simulink model "Torque_Control"  (R2022a)
settings: Solver=FixedStepAuto  StartTime=0.0  StopTime=10.0  RelTol=1e-3
libraries: simulink x9, eeGeneralControl x3
(part 4 of 6)

== system Torque_Control/VDC/Vehicle Dynamics Control Modes/VDC Complete/Optimization SKF & CKF/Subsystem /SKF ==
  Derivative : Inport
  "SKF_Initial " : Inport  Port=2
  SKF_prev : Inport  Port=3
  Cte_SKF : Inport  Port=4
  Action Port : ActionPort  ActionPortLabel=if { }
  Display : Display
  If : If  IfExpression=u1 >=900  ElseIfExpressions=u1 < 900  ShowElse=off
  Merge : Merge
  No spin : Subsystem  TreatAsAtomicUnit=on
  Saturation : Saturate  UpperLimit=1  LowerLimit=0.3
  Spin : Subsystem  TreatAsAtomicUnit=on
  SKF_act : Outport  VectorParamsAs1DForOutWhenUnconnected=off
  wires:
  Merge/1 -> Saturation/1
  Derivative/1 -> If/1, Display/1
  Spin/1(SKF_act1) -> Merge/2
  "SKF_Initial "/1 -> No spin/1(SKF_Initial), Spin/1(SKF_Initial)
  No spin/1(SKF_act0) -> Merge/1
  If/2 -> No spin/Action
  SKF_prev/1 -> No spin/2(SKF_prev), Spin/2(SKF_prev)
  Cte_SKF/1 -> No spin/3(Cte_SKF), Spin/3(Cte_SKF)
  Saturation/1 -> SKF_act/1
  If/1 -> Spin/Action

== system Torque_Control/VDC/Vehicle Dynamics Control Modes/VDC without Longitudinal/Constraints/Acelerating and braking without Regenerative/If Action 1 ==
  Trans_max_dynamic : Inport
  Action Port : ActionPort  ActionPortLabel=if { }
  Trans_limit : Outport  VectorParamsAs1DForOutWhenUnconnected=off
  wires:
  Trans_max_dynamic/1 -> Trans_limit/1

== system Torque_Control/VDC/Vehicle Dynamics Control Modes/VDC without Longitudinal/Constraints/Acelerating and braking without Regenerative/If Action 2 ==
  "Trans_max_static " : Inport
  Action Port : ActionPort  ActionPortLabel=else { }
  Trans_limit : Outport  VectorParamsAs1DForOutWhenUnconnected=off
  wires:
  "Trans_max_static "/1 -> Trans_limit/1

== system Torque_Control/VDC/Vehicle Dynamics Control Modes/VDC without Longitudinal/Constraints/Acelerating and braking without Regenerative/Momentum Z scaled ==
  Tq_RR_Lim : Inport
  Tq_RL_Lim : Inport  Port=2
  Tq_RR_wc : Inport  Port=3
  Tq_RL_wc : Inport  Port=4
  MATLAB Function : MATLAB Function  TreatAsAtomicUnit=on
  TQ_RR : Outport  VectorParamsAs1DForOutWhenUnconnected=off
  TQ_RL : Outport  Port=2  VectorParamsAs1DForOutWhenUnconnected=off
  wires:
  Tq_RL_Lim/1 -> MATLAB Function/2(tq_RL_lim)
  Tq_RR_Lim/1 -> MATLAB Function/1(tq_RR_lim)
  Tq_RR_wc/1 -> MATLAB Function/3(tq_RR_wc)
  Tq_RL_wc/1 -> MATLAB Function/4(tq_RL_wc)
  MATLAB Function/1(TQ_RR) -> TQ_RR/1
  MATLAB Function/2(TQ_RL) -> TQ_RL/1

== system Torque_Control/VDC/Vehicle Dynamics Control Modes/VDC without Longitudinal/Optimization SKF & CKF/Subsystem /CKF ==
  Derivative : Inport
  CKF_Initial : Inport  Port=2
  "CKF_prev " : Inport  Port=3
  Cte_CKF : Inport  Port=4
  If1 : If  IfExpression=u1 >= 900  ElseIfExpressions=u1 < 900  ShowElse=off
  Merge : Merge
  No spin : Subsystem  TreatAsAtomicUnit=on
  Saturation : Saturate  UpperLimit=1  LowerLimit=0.3
  "Spin " : Subsystem  TreatAsAtomicUnit=on
  "CKF_act " : Outport  VectorParamsAs1DForOutWhenUnconnected=off
  wires:
  Merge/1 -> Saturation/1
  "CKF_prev "/1 -> "Spin "/1(CKF_prev), No spin/2(CKF_prev)
  Derivative/1 -> If1/1
  Cte_CKF/1 -> No spin/3(Cte_CKF), "Spin "/3(Cte_CKF)
  "Spin "/1("CKF_act1 ") -> Merge/2
  Saturation/1 -> "CKF_act "/1
  CKF_Initial/1 -> "Spin "/2("CKF_Initial "), No spin/1(CKF_Initial)
  If1/2 -> No spin/Action
  No spin/1(CKF_act0) -> Merge/1
  If1/1 -> "Spin "/Action

== system Torque_Control/VDC/Vehicle Dynamics Control Modes/Steering TV with TC/Optimization SKF & CKF/Subsystem /CKF/No spin ==
  CKF_Initial : Inport
  CKF_prev : Inport  Port=2
  Cte_CKF : Inport  Port=3
  Action Port : ActionPort  ActionPortLabel=elseif { }
  Display : Display
  Display1 : Display
  MATLAB Function : MATLAB Function  TreatAsAtomicUnit=on
  Switch : Switch  Criteria=u2 > Threshold  SaturateOnIntegerOverflow=off  InputSameDT=off
  CKF_act0 : Outport  VectorParamsAs1DForOutWhenUnconnected=off
  wires:
  CKF_Initial/1 -> MATLAB Function/2(CKF_Initial), Switch/3
  MATLAB Function/1(CKF_act0) -> CKF_act0/1, Display1/1
  CKF_prev/1 -> Switch/1, Switch/2
  Switch/1 -> Display/1, MATLAB Function/1(CKF_prev)
  Cte_CKF/1 -> MATLAB Function/3(Cte_CKF)

== system Torque_Control/VDC/Vehicle Dynamics Control Modes/Steering TV with TC/Optimization SKF & CKF/Subsystem /CKF/Spin  ==
  CKF_prev : Inport
  "CKF_Initial " : Inport  Port=2
  Cte_CKF : Inport  Port=3
  Action Port : ActionPort  ActionPortLabel=if { }
  Constant : Constant
  Display : Display
  Display1 : Display
  MATLAB Function : MATLAB Function  TreatAsAtomicUnit=on
  Product : Product
  Scope : Scope
  Switch : Switch  Threshold=0.9  SaturateOnIntegerOverflow=off  InputSameDT=off
  Switch1 : Switch  Criteria=u2 > Threshold  SaturateOnIntegerOverflow=off  InputSameDT=off
  "CKF_act1 " : Outport  VectorParamsAs1DForOutWhenUnconnected=off
  wires:
  MATLAB Function/1(CKF_act1) -> Display1/1, "CKF_act1 "/1
  Product/1 -> Display/1, MATLAB Function/2(CKF_prev)
  "CKF_Initial "/1 -> Switch1/3, MATLAB Function/1(CKF_Initial)
  Cte_CKF/1 -> Switch/2, Switch/1
  Constant/1 -> Switch/3
  Switch/1 -> Product/2
  Switch1/1 -> Scope/1, Product/1
  CKF_prev/1 -> Switch1/2, Switch1/1

== system Torque_Control/VDC/Vehicle Dynamics Control Modes/Steering TV with TC/Optimization SKF & CKF/Subsystem /SKF/No spin ==
  SKF_Initial : Inport
  SKF_prev : Inport  Port=2
  Cte_SKF : Inport  Port=3
  Action Port : ActionPort  ActionPortLabel=elseif { }
  Display : Display
  Display1 : Display
  MATLAB Function : MATLAB Function  TreatAsAtomicUnit=on
  Switch : Switch  Criteria=u2 > Threshold  SaturateOnIntegerOverflow=off  InputSameDT=off
  SKF_act0 : Outport  VectorParamsAs1DForOutWhenUnconnected=off
  wires:
  SKF_Initial/1 -> MATLAB Function/2(SKF_Initial), Switch/3
  MATLAB Function/1(SKF_act0) -> Display/1, SKF_act0/1
  Switch/1 -> MATLAB Function/1(SKF_prev)
  SKF_prev/1 -> Switch/1, Switch/2, Display1/1
  Cte_SKF/1 -> MATLAB Function/3(Cte_SKF)

== system Torque_Control/VDC/Vehicle Dynamics Control Modes/Steering TV with TC/Optimization SKF & CKF/Subsystem /SKF/Spin ==
  SKF_Initial : Inport
  SKF_prev : Inport  Port=2
  Cte_SKF : Inport  Port=3
  Action Port : ActionPort  ActionPortLabel=if { }
  Constant : Constant
  MATLAB Function : MATLAB Function  TreatAsAtomicUnit=on
  Product : Product
  Switch : Switch  Threshold=0.9  SaturateOnIntegerOverflow=off  InputSameDT=off
  Switch1 : Switch  Criteria=u2 > Threshold  SaturateOnIntegerOverflow=off  InputSameDT=off
  SKF_act1 : Outport  VectorParamsAs1DForOutWhenUnconnected=off
  wires:
  SKF_Initial/1 -> Switch1/3, MATLAB Function/1(SKF_Initial)
  Product/1 -> MATLAB Function/2(SKF_prev)
  MATLAB Function/1(SKF_act1) -> SKF_act1/1
  Switch/1 -> Product/2
  Cte_SKF/1 -> Switch/2, Switch/1
  Constant/1 -> Switch/3
  SKF_prev/1 -> Switch1/2, Switch1/1
  Switch1/1 -> Product/1

== system Torque_Control/VDC/Vehicle Dynamics Control Modes/VDC Complete/Optimization SKF & CKF/Subsystem /CKF/No spin ==
  CKF_Initial : Inport
  CKF_prev : Inport  Port=2
  Cte_CKF : Inport  Port=3
  Action Port : ActionPort  ActionPortLabel=elseif { }
  MATLAB Function1 : MATLAB Function  TreatAsAtomicUnit=on
  Switch1 : Switch  Criteria=u2 > Threshold  SaturateOnIntegerOverflow=off  InputSameDT=off
  CKF_act0 : Outport  VectorParamsAs1DForOutWhenUnconnected=off
  wires:
  Cte_CKF/1 -> MATLAB Function1/3(Cte_CKF)
  Switch1/1 -> MATLAB Function1/1(CKF_prev)
  CKF_Initial/1 -> Switch1/3, MATLAB Function1/2(CKF_Initial)
  CKF_prev/1 -> Switch1/2, Switch1/1
  MATLAB Function1/1(CKF_act0) -> CKF_act0/1

== system Torque_Control/VDC/Vehicle Dynamics Control Modes/VDC Complete/Optimization SKF & CKF/Subsystem /CKF/Spin  ==
  CKF_prev : Inport
  "CKF_Initial " : Inport  Port=2
  Cte_CKF : Inport  Port=3
  Action Port : ActionPort  ActionPortLabel=if { }
  Constant : Constant
  MATLAB Function : MATLAB Function  TreatAsAtomicUnit=on
  Product : Product
  Switch : Switch  Criteria=u2 > Threshold  Threshold=0.9  SaturateOnIntegerOverflow=off  InputSameDT=off
  Switch1 : Switch  Criteria=u2 > Threshold  SaturateOnIntegerOverflow=off  InputSameDT=off
  "CKF_act1 " : Outport  VectorParamsAs1DForOutWhenUnconnected=off
  wires:
  MATLAB Function/1(CKF_act1) -> "CKF_act1 "/1
  Product/1 -> MATLAB Function/2(CKF_prev)
  "CKF_Initial "/1 -> Switch1/3, MATLAB Function/1(CKF_Initial)
  Cte_CKF/1 -> Switch/2, Switch/1
  Constant/1 -> Switch/3
  Switch/1 -> Product/2
  Switch1/1 -> Product/1
  CKF_prev/1 -> Switch1/2, Switch1/1

== system Torque_Control/VDC/Vehicle Dynamics Control Modes/VDC Complete/Optimization SKF & CKF/Subsystem /SKF/No spin ==
  SKF_Initial : Inport
  SKF_prev : Inport  Port=2
  Cte_SKF : Inport  Port=3
  Action Port : ActionPort  ActionPortLabel=elseif { }
  MATLAB Function : MATLAB Function  TreatAsAtomicUnit=on
  Switch1 : Switch  Criteria=u2 > Threshold  SaturateOnIntegerOverflow=off  InputSameDT=off
  SKF_act0 : Outport  VectorParamsAs1DForOutWhenUnconnected=off
  wires:
  SKF_Initial/1 -> MATLAB Function/2(SKF_Initial), Switch1/3
  Switch1/1 -> MATLAB Function/1(SKF_prev)
  SKF_prev/1 -> Switch1/1, Switch1/2
  MATLAB Function/1(SKF_act0) -> SKF_act0/1
  Cte_SKF/1 -> MATLAB Function/3(Cte_SKF)

== system Torque_Control/VDC/Vehicle Dynamics Control Modes/VDC Complete/Optimization SKF & CKF/Subsystem /SKF/Spin ==
  SKF_Initial : Inport
  SKF_prev : Inport  Port=2
  Cte_SKF : Inport  Port=3
  Action Port : ActionPort  ActionPortLabel=if { }
  Constant : Constant
  MATLAB Function : MATLAB Function  TreatAsAtomicUnit=on
  Product : Product
  Switch : Switch  Threshold=0.9  SaturateOnIntegerOverflow=off  InputSameDT=off
  Switch1 : Switch  Criteria=u2 > Threshold  SaturateOnIntegerOverflow=off  InputSameDT=off
  SKF_act1 : Outport  VectorParamsAs1DForOutWhenUnconnected=off
  wires:
  SKF_Initial/1 -> Switch1/3, MATLAB Function/1(SKF_Initial)
  Product/1 -> MATLAB Function/2(SKF_prev)
  MATLAB Function/1(SKF_act1) -> SKF_act1/1
  Switch/1 -> Product/2
  Cte_SKF/1 -> Switch/2, Switch/1
  Constant/1 -> Switch/3
  Switch1/1 -> Product/1
  SKF_prev/1 -> Switch1/2, Switch1/1

== system Torque_Control/VDC/Vehicle Dynamics Control Modes/VDC without Longitudinal/Optimization SKF & CKF/Subsystem /CKF/No spin ==
  CKF_Initial : Inport
  CKF_prev : Inport  Port=2
  Cte_CKF : Inport  Port=3
  Action Port : ActionPort  ActionPortLabel=elseif { }
  MATLAB Function : MATLAB Function  TreatAsAtomicUnit=on
  Switch1 : Switch  Criteria=u2 > Threshold  SaturateOnIntegerOverflow=off  InputSameDT=off
  CKF_act0 : Outport  VectorParamsAs1DForOutWhenUnconnected=off
  wires:
  Cte_CKF/1 -> MATLAB Function/3(Cte_CKF)
  Switch1/1 -> MATLAB Function/1(CKF_prev)
  CKF_Initial/1 -> Switch1/3, MATLAB Function/2(CKF_Initial)
  CKF_prev/1 -> Switch1/1, Switch1/2
  MATLAB Function/1(CKF_act0) -> CKF_act0/1

== system Torque_Control/VDC/Vehicle Dynamics Control Modes/VDC without Longitudinal/Optimization SKF & CKF/Subsystem /CKF/Spin  ==
  CKF_prev : Inport
  "CKF_Initial " : Inport  Port=2
  Cte_CKF : Inport  Port=3
  Action Port : ActionPort  ActionPortLabel=if { }
  Constant : Constant
  MATLAB Function : MATLAB Function  TreatAsAtomicUnit=on
  Product : Product
  Switch : Switch  Threshold=0.9  SaturateOnIntegerOverflow=off  InputSameDT=off
  Switch1 : Switch  Criteria=u2 > Threshold  SaturateOnIntegerOverflow=off  InputSameDT=off
  "CKF_act1 " : Outport  VectorParamsAs1DForOutWhenUnconnected=off
  wires:
  MATLAB Function/1(CKF_act1) -> "CKF_act1 "/1
  Product/1 -> MATLAB Function/2(CKF_prev)
  "CKF_Initial "/1 -> Switch1/3, MATLAB Function/1(CKF_Initial)
  Cte_CKF/1 -> Switch/2, Switch/1
  Constant/1 -> Switch/3
  Switch/1 -> Product/2
  CKF_prev/1 -> Switch1/2, Switch1/1
  Switch1/1 -> Product/1

== matlab function Torque_Control/VDC/Vehicle Dynamics Control Modes/VDC without Longitudinal/Kamm Circle Lateral/Kamm_Circle LatD ==
  data: Fx_R output; Fz_R input; Fz_L input; Fy input; Fx_L output
function [Fx_R,Fx_L]= kamm_search_Fx(Fz_R,Fz_L,Fy)
kamm_data = zeros(17,32);
kamm_data(1,1) = NaN;
kamm_data(1,2) = 0;
kamm_data(1,3) = 100;
kamm_data(1,4) = 200;
kamm_data(1,5) = 300;
kamm_data(1,6) = 400;
kamm_data(1,7) = 500;
kamm_data(1,8) = 600;
kamm_data(1,9) = 700;
kamm_data(1,10) = 800;
kamm_data(1,11) = 900;
kamm_data(1,12) = 1000;
kamm_data(1,13) = 1100;
kamm_data(1,14) = 1200;
kamm_data(1,15) = 1300;
kamm_data(1,16) = 1400;
kamm_data(1,17) = 1500;
kamm_data(1,18) = 1600;
kamm_data(1,19) = 1700;
kamm_data(1,20) = 1800;
kamm_data(1,21) = 1900;
kamm_data(1,22) = 2000;
kamm_data(1,23) = 2100;
kamm_data(1,24) = 2200;
kamm_data(1,25) = 2300;
kamm_data(1,26) = 2400;
kamm_data(1,27) = 2500;
kamm_data(1,28) = 2600;
kamm_data(1,29) = 2700;
kamm_data(1,30) = 2800;
kamm_data(1,31) = 2900;
kamm_data(1,32) = 3000;
kamm_data(2,1) = 0;
kamm_data(2,2) = 0;
kamm_data(2,3) = NaN;
kamm_data(2,4) = NaN;
kamm_data(2,5) = NaN;
kamm_data(2,6) = NaN;
kamm_data(2,7) = NaN;
kamm_data(2,8) = NaN;
kamm_data(2,9) = NaN;
kamm_data(2,10) = NaN;
kamm_data(2,11) = NaN;
kamm_data(2,12) = NaN;
kamm_data(2,13) = NaN;
kamm_data(2,14) = NaN;
kamm_data(2,15) = NaN;
kamm_data(2,16) = NaN;
kamm_data(2,17) = NaN;
kamm_data(2,18) = NaN;
kamm_data(2,19) = NaN;
kamm_data(2,20) = NaN;
kamm_data(2,21) = NaN;
kamm_data(2,22) = NaN;
kamm_data(2,23) = NaN;
kamm_data(2,24) = NaN;
kamm_data(2,25) = NaN;
kamm_data(2,26) = NaN;
kamm_data(2,27) = NaN;
kamm_data(2,28) = NaN;
kamm_data(2,29) = NaN;
kamm_data(2,30) = NaN;
kamm_data(2,31) = NaN;
kamm_data(2,32) = NaN;
kamm_data(3,1) = 100;
kamm_data(3,2) = 350;
kamm_data(3,3) = 340;
kamm_data(3,4) = 156;
kamm_data(3,5) = NaN;
kamm_data(3,6) = NaN;
kamm_data(3,7) = NaN;
kamm_data(3,8) = NaN;
kamm_data(3,9) = NaN;
kamm_data(3,10) = NaN;
kamm_data(3,11) = NaN;
kamm_data(3,12) = NaN;
kamm_data(3,13) = NaN;
kamm_data(3,14) = NaN;
kamm_data(3,15) = NaN;
kamm_data(3,16) = NaN;
kamm_data(3,17) = NaN;
kamm_data(3,18) = NaN;
kamm_data(3,19) = NaN;
kamm_data(3,20) = NaN;
kamm_data(3,21) = NaN;
kamm_data(3,22) = NaN;
kamm_data(3,23) = NaN;
kamm_data(3,24) = NaN;
kamm_data(3,25) = NaN;
kamm_data(3,26) = NaN;
kamm_data(3,27) = NaN;
kamm_data(3,28) = NaN;
kamm_data(3,29) = NaN;
kamm_data(3,30) = NaN;
kamm_data(3,31) = NaN;
kamm_data(3,32) = NaN;
kamm_data(4,1) = 200;
kamm_data(4,2) = 688;
kamm_data(4,3) = 676;
kamm_data(4,4) = 654;
kamm_data(4,5) = 573;
kamm_data(4,6) = 269;
kamm_data(4,7) = NaN;
kamm_data(4,8) = NaN;
kamm_data(4,9) = NaN;
kamm_data(4,10) = NaN;
kamm_data(4,11) = NaN;
kamm_data(4,12) = NaN;
kamm_data(4,13) = NaN;
kamm_data(4,14) = NaN;
kamm_data(4,15) = NaN;
kamm_data(4,16) = NaN;
kamm_data(4,17) = NaN;
kamm_data(4,18) = NaN;
kamm_data(4,19) = NaN;
kamm_data(4,20) = NaN;
kamm_data(4,21) = NaN;
kamm_data(4,22) = NaN;
kamm_data(4,23) = NaN;
kamm_data(4,24) = NaN;
kamm_data(4,25) = NaN;
kamm_data(4,26) = NaN;
kamm_data(4,27) = NaN;
kamm_data(4,28) = NaN;
kamm_data(4,29) = NaN;
kamm_data(4,30) = NaN;
kamm_data(4,31) = NaN;
kamm_data(4,32) = NaN;
kamm_data(5,1) = 300;
kamm_data(5,2) = 1002;
kamm_data(5,3) = 994;
kamm_data(5,4) = 982;
kamm_data(5,5) = 959;
kamm_data(5,6) = 888;
kamm_data(5,7) = 694;
kamm_data(5,8) = 345;
kamm_data(5,9) = NaN;
kamm_data(5,10) = NaN;
kamm_data(5,11) = NaN;
kamm_data(5,12) = NaN;
kamm_data(5,13) = NaN;
kamm_data(5,14) = NaN;
kamm_data(5,15) = NaN;
kamm_data(5,16) = NaN;
kamm_data(5,17) = NaN;
kamm_data(5,18) = NaN;
kamm_data(5,19) = NaN;
kamm_data(5,20) = NaN;
kamm_data(5,21) = NaN;
kamm_data(5,22) = NaN;
kamm_data(5,23) = NaN;
kamm_data(5,24) = NaN;
kamm_data(5,25) = NaN;
kamm_data(5,26) = NaN;
kamm_data(5,27) = NaN;
kamm_data(5,28) = NaN;
kamm_data(5,29) = NaN;
kamm_data(5,30) = NaN;
kamm_data(5,31) = NaN;
kamm_data(5,32) = NaN;
kamm_data(6,1) = 400;
kamm_data(6,2) = 1295;
kamm_data(6,3) = 1288;
kamm_data(6,4) = 1280;
kamm_data(6,5) = 1263;
kamm_data(6,6) = 1235;
kamm_data(6,7) = 1168;
kamm_data(6,8) = 1001;
kamm_data(6,9) = 740;
kamm_data(6,10) = 389;
kamm_data(6,11) = NaN;
kamm_data(6,12) = NaN;
kamm_data(6,13) = NaN;
kamm_data(6,14) = NaN;
kamm_data(6,15) = NaN;
kamm_data(6,16) = NaN;
kamm_data(6,17) = NaN;
kamm_data(6,18) = NaN;
kamm_data(6,19) = NaN;
kamm_data(6,20) = NaN;
kamm_data(6,21) = NaN;
kamm_data(6,22) = NaN;
kamm_data(6,23) = NaN;
kamm_data(6,24) = NaN;
kamm_data(6,25) = NaN;
kamm_data(6,26) = NaN;
kamm_data(6,27) = NaN;
kamm_data(6,28) = NaN;
kamm_data(6,29) = NaN;
kamm_data(6,30) = NaN;
kamm_data(6,31) = NaN;
kamm_data(6,32) = NaN;
kamm_data(7,1) = 500;
kamm_data(7,2) = 1536;
kamm_data(7,3) = 1529;
kamm_data(7,4) = 1521;
kamm_data(7,5) = 1509;
kamm_data(7,6) = 1491;
kamm_data(7,7) = 1459;
kamm_data(7,8) = 1395;
kamm_data(7,9) = 1230;
kamm_data(7,10) = 1032;
kamm_data(7,11) = 760;
kamm_data(7,12) = 411;
kamm_data(7,13) = NaN;
kamm_data(7,14) = NaN;
kamm_data(7,15) = NaN;
kamm_data(7,16) = NaN;
kamm_data(7,17) = NaN;
kamm_data(7,18) = NaN;
kamm_data(7,19) = NaN;
kamm_data(7,20) = NaN;
kamm_data(7,21) = NaN;
kamm_data(7,22) = NaN;
kamm_data(7,23) = NaN;
kamm_data(7,24) = NaN;
kamm_data(7,25) = NaN;
kamm_data(7,26) = NaN;
kamm_data(7,27) = NaN;
kamm_data(7,28) = NaN;
kamm_data(7,29) = NaN;
kamm_data(7,30) = NaN;
kamm_data(7,31) = NaN;
kamm_data(7,32) = NaN;
kamm_data(8,1) = 600;
kamm_data(8,2) = 1745;
kamm_data(8,3) = 1737;
kamm_data(8,4) = 1729;
kamm_data(8,5) = 1721;
kamm_data(8,6) = 1704;
kamm_data(8,7) = 1686;
kamm_data(8,8) = 1649;
kamm_data(8,9) = 1585;
kamm_data(8,10) = 1455;
kamm_data(8,11) = 1270;
kamm_data(8,12) = 1038;
kamm_data(8,13) = 756;
kamm_data(8,14) = 419;
kamm_data(8,15) = NaN;
kamm_data(8,16) = NaN;
kamm_data(8,17) = NaN;
kamm_data(8,18) = NaN;
kamm_data(8,19) = NaN;
kamm_data(8,20) = NaN;
kamm_data(8,21) = NaN;
kamm_data(8,22) = NaN;
kamm_data(8,23) = NaN;
kamm_data(8,24) = NaN;
kamm_data(8,25) = NaN;
kamm_data(8,26) = NaN;
kamm_data(8,27) = NaN;
kamm_data(8,28) = NaN;
kamm_data(8,29) = NaN;
kamm_data(8,30) = NaN;
kamm_data(8,31) = NaN;
kamm_data(8,32) = NaN;
kamm_data(9,1) = 700;
kamm_data(9,2) = 1964;
kamm_data(9,3) = 1956;
kamm_data(9,4) = 1948;
kamm_data(9,5) = 1940;
kamm_data(9,6) = 1926;
kamm_data(9,7) = 1909;
kamm_data(9,8) = 1884;
kamm_data(9,9) = 1848;
kamm_data(9,10) = 1777;
kamm_data(9,11) = 1656;
kamm_data(9,12) = 1484;
kamm_data(9,13) = 1278;
kamm_data(9,14) = 1029;
kamm_data(9,15) = 742;
kamm_data(9,16) = 416;
kamm_data(9,17) = NaN;
kamm_data(9,18) = NaN;
kamm_data(9,19) = NaN;
kamm_data(9,20) = NaN;
kamm_data(9,21) = NaN;
kamm_data(9,22) = NaN;
kamm_data(9,23) = NaN;
kamm_data(9,24) = NaN;
kamm_data(9,25) = NaN;
kamm_data(9,26) = NaN;
kamm_data(9,27) = NaN;
kamm_data(9,28) = NaN;
kamm_data(9,29) = NaN;
kamm_data(9,30) = NaN;
kamm_data(9,31) = NaN;
kamm_data(9,32) = NaN;
kamm_data(10,1) = 800;
kamm_data(10,2) = 2212;
kamm_data(10,3) = 2204;
kamm_data(10,4) = 2195;
kamm_data(10,5) = 2187;
kamm_data(10,6) = 2175;
kamm_data(10,7) = 2158;
kamm_data(10,8) = 2141;
kamm_data(10,9) = 2107;
kamm_data(10,10) = 2063;
kamm_data(10,11) = 1990;
kamm_data(10,12) = 1868;
kamm_data(10,13) = 1704;
kamm_data(10,14) = 1505;
kamm_data(10,15) = 1275;
kamm_data(10,16) = 1018;
kamm_data(10,17) = 730;
kamm_data(10,18) = 404;
kamm_data(10,19) = NaN;
kamm_data(10,20) = NaN;
kamm_data(10,21) = NaN;
kamm_data(10,22) = NaN;
kamm_data(10,23) = NaN;
kamm_data(10,24) = NaN;
kamm_data(10,25) = NaN;
kamm_data(10,26) = NaN;
kamm_data(10,27) = NaN;
kamm_data(10,28) = NaN;
kamm_data(10,29) = NaN;
kamm_data(10,30) = NaN;
kamm_data(10,31) = NaN;
kamm_data(10,32) = NaN;
kamm_data(11,1) = 900;
kamm_data(11,2) = 2465;
kamm_data(11,3) = 2456;
kamm_data(11,4) = 2448;
kamm_data(11,5) = 2439;
kamm_data(11,6) = 2428;
kamm_data(11,7) = 2411;
kamm_data(11,8) = 2394;
kamm_data(11,9) = 2367;
kamm_data(11,10) = 2333;
kamm_data(11,11) = 2279;
kamm_data(11,12) = 2200;
kamm_data(11,13) = 2081;
kamm_data(11,14) = 1921;
kamm_data(11,15) = 1729;
kamm_data(11,16) = 1512;
kamm_data(11,17) = 1268;
kamm_data(11,18) = 1002;
kamm_data(11,19) = 711;
kamm_data(11,20) = 345;
kamm_data(11,21) = NaN;
kamm_data(11,22) = NaN;
kamm_data(11,23) = NaN;
kamm_data(11,24) = NaN;
kamm_data(11,25) = NaN;
kamm_data(11,26) = NaN;
kamm_data(11,27) = NaN;
kamm_data(11,28) = NaN;
kamm_data(11,29) = NaN;
kamm_data(11,30) = NaN;
kamm_data(11,31) = NaN;
kamm_data(11,32) = NaN;
kamm_data(12,1) = 1000;
kamm_data(12,2) = 2684;
kamm_data(12,3) = 2675;
kamm_data(12,4) = 2666;
kamm_data(12,5) = 2657;
kamm_data(12,6) = 2647;
kamm_data(12,7) = 2629;
kamm_data(12,8) = 2612;
kamm_data(12,9) = 2592;
kamm_data(12,10) = 2558;
kamm_data(12,11) = 2520;
kamm_data(12,12) = 2462;
kamm_data(12,13) = 2378;
kamm_data(12,14) = 2262;
kamm_data(12,15) = 2119;
kamm_data(12,16) = 1940;
kamm_data(12,17) = 1737;
kamm_data(12,18) = 1508;
kamm_data(12,19) = 1259;
kamm_data(12,20) = 989;
kamm_data(12,21) = 680;
kamm_data(12,22) = 240;
kamm_data(12,23) = NaN;
kamm_data(12,24) = NaN;
kamm_data(12,25) = NaN;
kamm_data(12,26) = NaN;
kamm_data(12,27) = NaN;
kamm_data(12,28) = NaN;
kamm_data(12,29) = NaN;
kamm_data(12,30) = NaN;
kamm_data(12,31) = NaN;
kamm_data(12,32) = NaN;
kamm_data(13,1) = 1100;
kamm_data(13,2) = 2853;
kamm_data(13,3) = 2843;
kamm_data(13,4) = 2833;
kamm_data(13,5) = 2822;
kamm_data(13,6) = 2811;
kamm_data(13,7) = 2795;
kamm_data(13,8) = 2775;
kamm_data(13,9) = 2755;
kamm_data(13,10) = 2728;
kamm_data(13,11) = 2693;
kamm_data(13,12) = 2651;
kamm_data(13,13) = 2591;
kamm_data(13,14) = 2510;
kamm_data(13,15) = 2412;
kamm_data(13,16) = 2282;
kamm_data(13,17) = 2124;
kamm_data(13,18) = 1940;
kamm_data(13,19) = 1735;
kamm_data(13,20) = 1504;
kamm_data(13,21) = 1250;
kamm_data(13,22) = 962;
kamm_data(13,23) = 608;
kamm_data(13,24) = 108;
kamm_data(13,25) = NaN;
kamm_data(13,26) = NaN;
kamm_data(13,27) = NaN;
kamm_data(13,28) = NaN;
kamm_data(13,29) = NaN;
kamm_data(13,30) = NaN;
kamm_data(13,31) = NaN;
kamm_data(13,32) = NaN;
kamm_data(14,1) = 1200;
kamm_data(14,2) = 2999;
kamm_data(14,3) = 2988;
kamm_data(14,4) = 2976;
kamm_data(14,5) = 2964;
kamm_data(14,6) = 2952;
kamm_data(14,7) = 2936;
kamm_data(14,8) = 2914;
kamm_data(14,9) = 2893;
kamm_data(14,10) = 2872;
kamm_data(14,11) = 2837;
kamm_data(14,12) = 2799;
kamm_data(14,13) = 2755;
kamm_data(14,14) = 2694;
kamm_data(14,15) = 2619;
kamm_data(14,16) = 2527;
kamm_data(14,17) = 2412;
kamm_data(14,18) = 2275;
kamm_data(14,19) = 2114;
kamm_data(14,20) = 1936;
kamm_data(14,21) = 1729;
kamm_data(14,22) = 1507;
kamm_data(14,23) = 1233;
kamm_data(14,24) = 896;
kamm_data(14,25) = 461;
kamm_data(14,26) = NaN;
kamm_data(14,27) = NaN;
kamm_data(14,28) = NaN;
kamm_data(14,29) = NaN;
kamm_data(14,30) = NaN;
kamm_data(14,31) = NaN;
kamm_data(14,32) = NaN;
kamm_data(15,1) = 1300;
kamm_data(15,2) = 3128;
kamm_data(15,3) = 3115;
kamm_data(15,4) = 3101;
kamm_data(15,5) = 3087;
kamm_data(15,6) = 3074;
kamm_data(15,7) = 3059;
kamm_data(15,8) = 3035;
kamm_data(15,9) = 3012;
kamm_data(15,10) = 2988;
kamm_data(15,11) = 2962;
kamm_data(15,12) = 2923;
kamm_data(15,13) = 2884;
kamm_data(15,14) = 2838;
kamm_data(15,15) = 2778;
kamm_data(15,16) = 2709;
kamm_data(15,17) = 2625;
kamm_data(15,18) = 2517;
kamm_data(15,19) = 2396;
kamm_data(15,20) = 2259;
kamm_data(15,21) = 2104;
kamm_data(15,22) = 1924;
kamm_data(15,23) = 1730;
kamm_data(15,24) = 1484;
kamm_data(15,25) = 1169;
kamm_data(15,26) = 772;
kamm_data(15,27) = 213;
kamm_data(15,28) = NaN;
kamm_data(15,29) = NaN;
kamm_data(15,30) = NaN;
kamm_data(15,31) = NaN;
kamm_data(15,32) = NaN;
kamm_data(16,1) = 1400;
kamm_data(16,2) = 3228;
kamm_data(16,3) = 3215;
kamm_data(16,4) = 3201;
kamm_data(16,5) = 3187;
kamm_data(16,6) = 3172;
kamm_data(16,7) = 3157;
kamm_data(16,8) = 3134;
kamm_data(16,9) = 3111;
kamm_data(16,10) = 3087;
kamm_data(16,11) = 3063;
kamm_data(16,12) = 3026;
kamm_data(16,13) = 2989;
kamm_data(16,14) = 2952;
kamm_data(16,15) = 2896;
kamm_data(16,16) = 2841;
kamm_data(16,17) = 2772;
kamm_data(16,18) = 2691;
kamm_data(16,19) = 2603;
kamm_data(16,20) = 2500;
kamm_data(16,21) = 2379;
kamm_data(16,22) = 2243;
kamm_data(16,23) = 2091;
kamm_data(16,24) = 1927;
kamm_data(16,25) = 1713;
kamm_data(16,26) = 1414;
kamm_data(16,27) = 1030;
kamm_data(16,28) = 553;
kamm_data(16,29) = NaN;
kamm_data(16,30) = NaN;
kamm_data(16,31) = NaN;
kamm_data(16,32) = NaN;
kamm_data(17,1) = 1500;
kamm_data(17,2) = 3327;
kamm_data(17,3) = 3312;
kamm_data(17,4) = 3296;
kamm_data(17,5) = 3280;
kamm_data(17,6) = 3263;
kamm_data(17,7) = 3247;
kamm_data(17,8) = 3223;
kamm_data(17,9) = 3198;
kamm_data(17,10) = 3173;
kamm_data(17,11) = 3147;
kamm_data(17,12) = 3116;
kamm_data(17,13) = 3078;
kamm_data(17,14) = 3040;
kamm_data(17,15) = 3001;
kamm_data(17,16) = 2947;
kamm_data(17,17) = 2893;
kamm_data(17,18) = 2828;
kamm_data(17,19) = 2756;
kamm_data(17,20) = 2670;
kamm_data(17,21) = 2576;
kamm_data(17,22) = 2471;
kamm_data(17,23) = 2353;
kamm_data(17,24) = 2228;
kamm_data(17,25) = 2100;
kamm_data(17,26) = 1921;
kamm_data(17,27) = 1649;
kamm_data(17,28) = 1278;
kamm_data(17,29) = 814;
kamm_data(17,30) = 217;
kamm_data(17,31) = NaN;
kamm_data(17,32) = NaN;

% DATA
Fz_data = kamm_data(2:end,1);
Fy_data = kamm_data(1,2:end);
Fx_data = kamm_data(2:end,2:end);
%% Encontrar la Fz en la data
% [mz,Mz] = dichotomic_search(Fz_data,Fz);
mz = 1;
Mz = length(Fz_data);
k = floor((mz+Mz)/2);
p = Mz-mz;
while p ~= 1;
    if Fz_R > Fz_data(k);
        mz = k;
    elseif Fz_R < Fz_data(k);
        Mz = k;
    end
    k = floor((Mz+mz)/2);
    p = Mz-mz;
    if Fz_R == Fz_data(Mz);
        p = 1;
        mz = Mz;
    elseif Fz_R == Fz_data(mz);
        p = 1;
        Mz = mz;
    elseif Fz_R == Fz_data(k);
        p = 1;
        Mz = k;
        mz = k;
    end  
end
%% Encontrar la FY en la data
% [my,My] = dichotomic_search(Fy_data,Fy);
my = 1;
My = length(Fy_data);
k = floor((my+My)/2);
p = My-my;
while p ~= 1;
    if Fy > Fy_data(k);
        my = k;
    elseif Fy < Fy_data(k);
        My = k;
    end
    k = floor((My+my)/2);
    p = My-my;
    if Fy == Fy_data(My);
        p = 1;
        my = My;
    elseif Fy == Fy_data(my);
        p = 1;
        My = my;
    elseif Fy == Fy_data(k);
        p = 1;
        My = k;
        my = k;
    end  
end
%% Restricciones
if Mz == mz && My ~= my % Existe el valor real de la Fz         % not OK
    Fy_MT = [Fy_data(my) Fy_data(My)]';
    Fx_MT = [Fx_data(mz,my) Fx_data(mz,My)]';
    a = polyfit(Fy_MT,Fx_MT,1);
    Fx_R = a(1)*Fy+a(2);
elseif Mz ~= mz && My == my % Existe el valor real de la Fy     % OK
    Fz_MT = [Fz_data(mz) Fz_data(Mz)]';
    Fx_MT = [Fx_data(mz,my) Fx_data(Mz,my)]';
    a = polyfit(Fz_MT,Fx_MT,1);
    Fx_R = a(1)*Fz_R+a(2);
elseif Mz == mz && My == my % Existen Fz y Fy       % OK           
    Fx_R = Fx_data(Mz,My);
else % No existe el valor de Fz ni Fy               % OK                   
    Fz_MT = [Fz_data(mz) Fz_data(mz) Fz_data(Mz) Fz_data(Mz)]'
    Fy_MT = [Fy_data(my) Fy_data(My) Fy_data(my) Fy_data(My)]'
    Fx_MT = [Fx_data(mz,my) Fx_data(mz,My) Fx_data(Mz,my) Fx_data(Mz,My)]'
    MT_solver = [ones(size(Fz_MT)) Fz_MT Fy_MT]
    a = MT_solver\Fx_MT;
    Fx_R = a(1)+a(2)*Fz_R+a(3)*Fy;
end

%%%%%%%%%%%%%%%%%%%%%%%%%%%%%%%%%%%%%%%%%%%%%%%%%%%
%% Encontrar la Fz en la data
% [mz,Mz] = dichotomic_search(Fz_data,Fz);
mz = 1;
Mz = length(Fz_data);
k = floor((mz+Mz)/2);
p = Mz-mz;
while p ~= 1;
    if Fz_L > Fz_data(k);
        mz = k;
    elseif Fz_L < Fz_data(k);
        Mz = k;
    end
    k = floor((Mz+mz)/2);
    p = Mz-mz;
    if Fz_L == Fz_data(Mz);
        p = 1;
        mz = Mz;
    elseif Fz_L == Fz_data(mz);
        p = 1;
        Mz = mz;
    elseif Fz_L == Fz_data(k);
        p = 1;
        Mz = k;
        mz = k;
    end  
end
%% Encontrar la FY en la data
% [my,My] = dichotomic_search(Fy_data,Fy);
my = 1;
My = length(Fy_data);
k = floor((my+My)/2);
p = My-my;
while p ~= 1;
    if Fy > Fy_data(k);
        my = k;
    elseif Fy < Fy_data(k);
        My = k;
    end
    k = floor((My+my)/2);
    p = My-my;
    if Fy == Fy_data(My);
        p = 1;
        my = My;
    elseif Fy == Fy_data(my);
        p = 1;
        My = my;
    elseif Fy == Fy_data(k);
        p = 1;
        My = k;
        my = k;
    end  
end
%% Restricciones
if Mz == mz && My ~= my % Existe el valor real de la Fz         % OK
    Fy_MT = [Fy_data(my) Fy_data(My)]';
    Fx_MT = [Fx_data(mz,my) Fx_data(mz,My)]';
    a = polyfit(Fy_MT,Fx_MT,1);
    Fx_L = a(1)*Fy+a(2);
elseif Mz ~= mz && My == my % Existe el valor real de la Fy     % OK
    Fz_MT = [Fz_data(mz) Fz_data(Mz)]';
    Fx_MT = [Fx_data(mz,my) Fx_data(Mz,my)]';
    a = polyfit(Fz_MT,Fx_MT,1);
    Fx_L = a(1)*Fz_L+a(2);
elseif Mz == mz && My == my % Existen Fz y Fy       % OK           
    Fx_L = Fx_data(Mz,My);
else % No existe el valor de Fz ni Fy               % OK                   
    Fz_MT = [Fz_data(mz) Fz_data(mz) Fz_data(Mz) Fz_data(Mz)]'
    Fy_MT = [Fy_data(my) Fy_data(My) Fy_data(my) Fy_data(My)]'
    Fx_MT = [Fx_data(mz,my) Fx_data(mz,My) Fx_data(Mz,my) Fx_data(Mz,My)]'
    MT_solver = [ones(size(Fz_MT)) Fz_MT Fy_MT]
    a = MT_solver\Fx_MT;
    Fx_L = a(1)+a(2)*Fz_L+a(3)*Fy;
end

== matlab function Torque_Control/VDC/Vehicle Dynamics Control Modes/VDC without Longitudinal/Constraints/Acelerating and braking without Regenerative/Momentum Z scaled/MATLAB Function ==
  data: tq_RR_lim input; TQ_RR output; tq_RL_lim input; tq_RR_wc input; tq_RL_wc input; TQ_RL output
function [TQ_RR,TQ_RL]= MomentumZ_scaled(tq_RR_lim,tq_RL_lim,tq_RR_wc,tq_RL_wc)
TQ_RR = 0;
TQ_RL = 0;
if tq_RR_lim == tq_RR_wc && tq_RL_lim == tq_RL_wc
    TQ_RR = tq_RR_lim;
    TQ_RL = tq_RL_lim;
else
    if tq_RR_wc > tq_RL_wc
        TQ_RR = tq_RR_lim;
        TQ_RL = (tq_RL_wc/tq_RR_wc)*tq_RR_lim;
    elseif tq_RR_wc < tq_RL_wc
        TQ_RR = (tq_RR_wc/tq_RL_wc)*tq_RL_lim;
        TQ_RL = tq_RL_lim;
    else
        TQ_RR = tq_RR_lim;
        TQ_RL = tq_RL_lim;
    end
end

== matlab function Torque_Control/VDC/Vehicle Dynamics Control Modes/VDC without Longitudinal/Constraints/Acelerating and braking without Regenerative/minimum value ==
  data: a input; min output; b input; c input
function min = fcn(a,b,c)
min = a;
if b < a;
    min = b;
end
if c < min;
    min = c;
end

== matlab function Torque_Control/VDC/Vehicle Dynamics Control Modes/VDC Complete/Longitudinal Dynamics/minimum value ==
  data: a input; min output; b input
function min = fcn(a,b)
min = a;
if b < a;
    min = b;
end

== matlab function Torque_Control/VDC/Vehicle Dynamics Control Modes/VDC without Longitudinal/Constraints/Acelerating and braking without Regenerative/minimum value1 ==
  data: a input; min output; b input; c input
function min = fcn(a,b,c)
min = a;
if b < a;
    min = b;
end
if c < min;
    min = c;
end

== matlab function Torque_Control/VDC/Vehicle Dynamics Control Modes/VDC without Longitudinal/Constraints/Braking with Regenerative/MATLAB Function ==
  data: MaxRegenTq input; RegTq_RR output; Tq_RR input; Tq_RL input; RegTq_RL output
function [RegTq_RR,RegTq_RL] = Regenerative_TV(MaxRegenTq,Tq_RR,Tq_RL)
RegTq_RR = 0;
RegTq_RL = 0;
if Tq_RR == 0 && Tq_RL == 0;
    RegTq_RR = 0;
    RegTq_RL = 0;
elseif Tq_RR ~= 0 && Tq_RL == 0;
    RegTq_RR = 0;
    RegTq_RL = Tq_RR;
elseif Tq_RR == 0 && Tq_RL ~= 0;
    RegTq_RR = Tq_RL;
    RegTq_RL = 0;
else
    if Tq_RR == Tq_RL;
        if Tq_RR >= MaxRegenTq;
            RegTq_RR = MaxRegenTq;
            RegTq_RL = MaxRegenTq;
        else
            RegTq_RR = Tq_RR;
            RegTq_RL = Tq_RL;
        end
    elseif Tq_RR > Tq_RL;
        if Tq_RR < MaxRegenTq 
            RegTq_RR = Tq_RL*Tq_RL/Tq_RR;
            RegTq_RL = Tq_RL;
        else
            RegTq_RR = MaxRegenTq*Tq_RL/Tq_RR;
            RegTq_RL = MaxRegenTq;
        end
    elseif Tq_RR < Tq_RL;
        if Tq_RL < MaxRegenTq 
            RegTq_RR = Tq_RR;
            RegTq_RL = Tq_RR*Tq_RR/Tq_RL;
        else
            RegTq_RR = MaxRegenTq;
            RegTq_RL = MaxRegenTq*Tq_RR/Tq_RL;
        end
    end
end

== matlab function Torque_Control/VDC/Vehicle Dynamics Control Modes/VDC Complete/Longitudinal Dynamics/MATLAB Function ==
  data: cte input; v input; value output
function value = switch_fcn(cte,v)
if v > 0 && v < 60000;
    value = v;
else
    value = cte;
end

== matlab function Torque_Control/VDC/Vehicle Dynamics Control Modes/VDC Complete/Longitudinal Dynamics/MATLAB Function1 ==
  data: cte input; v input; value output
function value = switch_fcn(cte,v)
if v > 0 && v < 60000;
    value = v;
else
    value = cte;
end

== matlab function Torque_Control/VDC/Vehicle Dynamics Control Modes/VDC Complete/Lateral Dynamics/MATLAB Function1 ==
  data: cte input; v input; value output
function value = switch_fcn(cte,v)
if v > 0 && v < 60000;
    value = v;
else
    value = cte;
end

== matlab function Torque_Control/VDC/Vehicle Dynamics Control Modes/VDC Complete/Lateral Dynamics/MATLAB Function2 ==
  data: cte input; v input; value output
function value = switch_fcn(cte,v)
if v > 0 && v < 60000;
    value = v;
else
    value = cte;
end

== matlab function Torque_Control/VDC/Vehicle Dynamics Control Modes/VDC Complete/Wheel_to_motor/MATLAB Function1 ==
  data: cte input; v input; value output
function value = switch_fcn(cte,v)
if v > 0;
    value = v;
else
    value = cte;
end

== matlab function Torque_Control/VDC/Vehicle Dynamics Control Modes/VDC Complete/Wheel_to_motor/MATLAB Function2 ==
  data: cte input; v input; value output
function value = switch_fcn(cte,v)
if v > 0;
    value = v;
else
    value = cte;
end

== matlab function Torque_Control/VDC/Vehicle Dynamics Control Modes/VDC without Longitudinal/Force to Tq/MATLAB Function2 ==
  data: cte input; v input; value output
function value = switch_fcn(cte,v)
if v > 0 && v < 60000;
    value = v;
else
    value = cte;
end

== matlab function Torque_Control/VDC/Vehicle Dynamics Control Modes/VDC without Longitudinal/Force to Tq/MATLAB Function1 ==
  data: cte input; v input; value output
function value = switch_fcn(cte,v)
if v > 0 && v < 60000;
    value = v;
else
    value = cte;
end
